simulink model "ZRD_Simulator"  (R2020a)
settings: Solver=VariableStepAuto  StartTime=0.0  StopTime=10.0  RelTol=1e-3
values from neighbouring files (symbols this model uses):
  a0 = 0    [ZRD_laengs.m]    (also in ZRD_laengsbewegung.m)
  g = 9.81    [ZRD_laengs.m]    (also in ZRD_laengsbewegung.m; ZRD_seitenbewegung.m)
  i_f = 0    [ZRD_laengs.m]    (also in ZRD_laengsbewegung.m)
  Ma = -0.3215    [ZRD_laengs.m]    (also in ZRD_laengsbewegung.m = 1)
  Mdf = -1.9727    [ZRD_laengs.m]    (also in ZRD_laengsbewegung.m = 1)
  Meta = -0.0967    [ZRD_laengs.m]    (also in ZRD_laengsbewegung.m = 1)
  Mq = 3.3984    [ZRD_laengs.m]    (also in ZRD_laengsbewegung.m = 1)
  Mv = 5.2744    [ZRD_laengs.m]    (also in ZRD_laengsbewegung.m = 1)
  V0 = 26.9962    [ZRD_laengs.m]    (also in ZRD_laengsbewegung.m = 30; ZRD_seitenbewegung.m = 30)
  Xa = -3.6481    [ZRD_laengs.m]    (also in ZRD_laengsbewegung.m = 1)
  Xdf = 2.8712    [ZRD_laengs.m]    (also in ZRD_laengsbewegung.m = 1)
  Xeta = -0.5580    (= -0.558)    [ZRD_laengs.m]    (also in ZRD_laengsbewegung.m = 1)
  Xv = 6.7118    [ZRD_laengs.m]    (also in ZRD_laengsbewegung.m = 1)
  Za = 9.9196    [ZRD_laengs.m]    (also in ZRD_laengsbewegung.m = 1)
  Zeta = 0.8461    [ZRD_laengs.m]    (also in ZRD_laengsbewegung.m = 1)
  Zv = -6.3420    (= -6.342)    [ZRD_laengs.m]    (also in ZRD_laengsbewegung.m = 1)
settings Model: Creator=Florian  LastModifiedBy=Florian

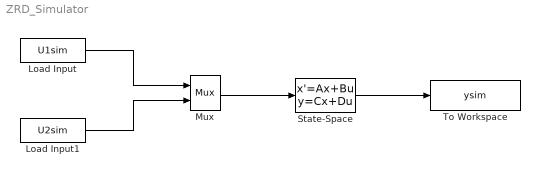
== system ZRD_Simulator ==
  Load Input : FromWorkspace  VariableName=U1sim  SampleTime=-1
  Load Input1 : FromWorkspace  VariableName=U2sim  SampleTime=-1
  Mux : Mux  Inputs=2
  State-Space : StateSpace  A=[Za/V0, 1, Zv/V0, 0; Ma, Mq, Mv, 0; Xa, 0, Xv, -g; -Za/V0, 0, -Zv/V0, 0]  B=[Zeta/V0, -Xdf/V0*sin(a0+i_f); Meta, Mdf; Xeta, Xdf*cos(a0+i_f); -Zeta/V0, Xdf/V0*sin(a0+i_f)]  C=eye(4,4);  D=zeros(4,2)  InitialCondition=zeros(1,4)
  To Workspace : ToWorkspace  VariableName=ysim  SampleTime=-1
  wires:
  Mux/1 -> State-Space/1
  State-Space/1 -> To Workspace/1
  Load Input/1 -> Mux/1
  Load Input1/1 -> Mux/2
